simulink subsystem "ElectricalThermalSystem"  (R2024b)
settings: Solver=VariableStepAuto  StartTime=0.0  StopTime=10.0  RelTol=1e-3
undefined symbols (not defined in the file): EnvAirTemp, PlantThrEstCmpPwr, PlntThrAirBpt, PlntThrAirCond, PlntThrAirCp, PlntThrAirCpBpt, PlntThrAirPrand, PlntThrAirRho, PlntThrAirVisc, PlntThrBattDCFlwRatio, PlntThrBattJacLen, PlntThrChArea, PlntThrChDia, PlntThrCoolCond, PlntThrCoolCp, PlntThrCoolCpBpt, PlntThrCoolPrand, PlntThrCoolRho, PlntThrCoolVisc, PlntThrDCJacLen, PlntThrEMJacLen, PlntThrEstCOPLut, PlntThrEstDTLut, PlntThrHeaterMaxPwr, PlntThrPmpDisp, PlntThrPmpHeadP, PlntThrPmpMaxSpd, PlntThrPmpMechEff, PlntThrPmpVolEff, PlntThrRadAirArea, PlntThrRadAirDh, PlntThrRadFanAreaFlw, PlntThrRadFlwCoef, PlntThrRadGapHeight, PlntThrRadLength, PlntThrRadNTubes, PlntThrRadTubeDh, PlntThrRadTubeHeight, PlntThrRadWidth
libraries: autolibutils x45
(part 1 of 4)
settings Model: ModifiedByFormat=The MathWorks, Inc.  Creator=The MathWorks, Inc.  LastModifiedBy=The MathWorks, Inc.
settings RTWCC: GPUComputeCapability=3.5  LargeConstantGeneration=WriteOnlyDNNConstantsToDataFiles

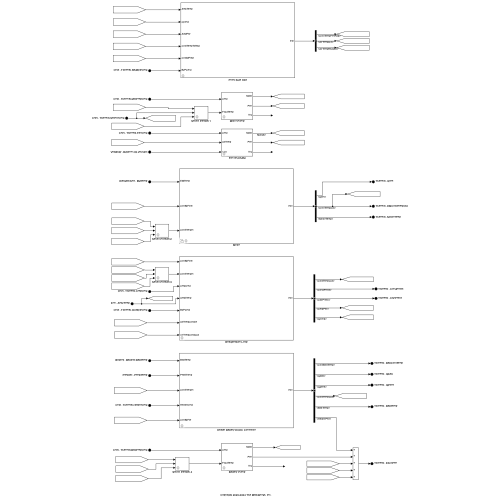
[thumbnail: Simulink's stored preview of the top-level diagram]
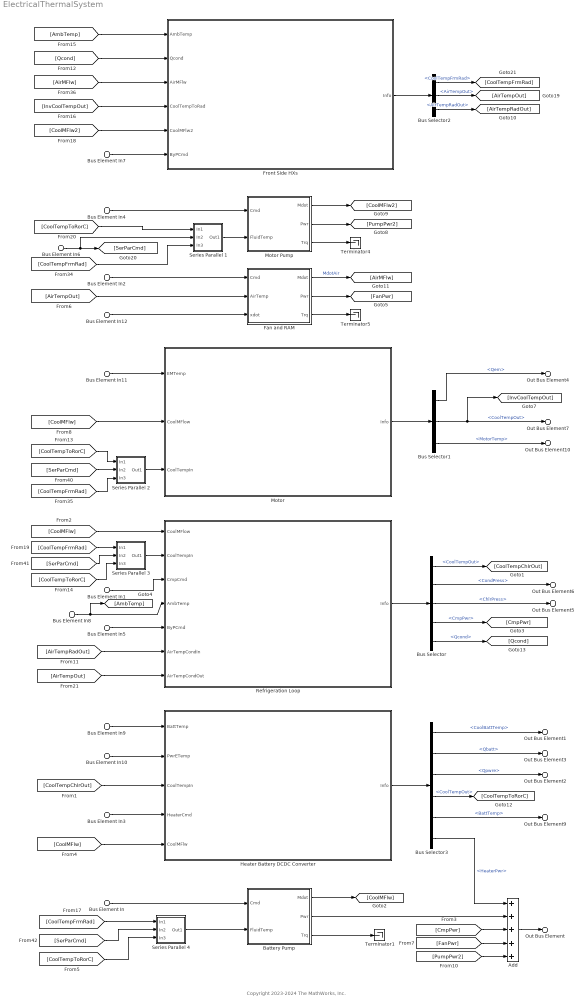
== system ElectricalThermalSystem ==
  note: Copyright 2023-2024 The MathWorks, Inc.
  Bus Element In : Inport  PortName=Cntrl  Element=Thermal.BattPmpCmd
  Bus Element In1 : Inport  PortName=Cntrl  Element=Thermal.CmpCmd
  Bus Element In2 : Inport  PortName=Cntrl  Element=Thermal.FanCmd
  Bus Element In3 : Inport  PortName=Cntrl  Element=Thermal.HeaterCmd
  Bus Element In4 : Inport  PortName=Cntrl  Element=Thermal.MotPmpCmd
  Bus Element In5 : Inport  PortName=Cntrl  Element=Thermal.ChlrByPCmd
  Bus Element In6 : Inport  PortName=Cntrl  Element=Thermal.SerParCmd
  Bus Element In7 : Inport  PortName=Cntrl  Element=Thermal.RadByPCmd
  Bus Element In8 : Inport  Port=2  PortName=Env  Element=AmbTemp
  Bus Element In9 : Inport  Port=3  PortName=Battery  Element=BattInfo.BattTemp
  Bus Element In10 : Inport  Port=4  PortName=PwrElec  Element=PwrETemp
  Bus Element In11 : Inport  Port=5  PortName=ElecMachine  Element=EMTemp
  Bus Element In12 : Inport  Port=6  PortName=VehBody  Element=BdyFrm.Cg.Vel.xdot
  Add : Sum  Inputs=+++++
  Battery Pump : Subsystem  mask{DispAng=PlntThrPmpDisp, MaxSpd=PlntThrPmpMaxSpd, VolEff=PlntThrPmpVolEff, MechEff=PlntThrPmpMechEff, HeadP=PlntThrPmpHeadP}
      mask prompts: DispAng "Displacement per revolution, DispAng [L/rev]"; MaxSpd "Max angular speed, MaxSpd [rpm]"; VolEff "Volumetric efficiency, VolEff [-]"; MechEff "Mechanical efficiency, MechEff [-]"; HeadP "Pressure gain, HeadP [Pa]"
      mask TypeOptions DispAng: Displ_LperRev/Value
      mask TypeOptions MaxSpd: MaxSpd_rpm/Value
      mask TypeOptions VolEff: VolumetricEfficiency/Value
      mask TypeOptions MechEff: MechanicalEfficiency/Value
      mask TypeOptions HeadP: PressGain_Pa/Value
      mask DialogControl DescTextVar Prompt: Battery Pump
      mask DialogControl ParameterGroupVar Prompt: Description
      mask DialogControl Control2 Prompt: Calculates the coolant mass flow through the loop that includes the battery and estimates the power and torque required by the pump.
      mask DialogControl Control3 Prompt: The mass flow calculation is an approximation for a positive displacement device.
      mask DialogControl Control4 Prompt: Mflw = Density*DispAng*Omega*VolEff
      mask DialogControl Control5 Prompt: Where:
      mask DialogControl Control6 Prompt: Mflw: mass flow
      mask DialogControl Control7 Prompt: DispAng: displacement/rotation angle
      mask DialogControl Control8 Prompt: Omega: angular speed
      mask DialogControl Control9 Prompt: VolEff: volumetric efficiency
      mask DialogControl Control10 Prompt: Torque = DispAng*MechEff*HeadP
      mask DialogControl Control11 Prompt: Where:
      mask DialogControl Control12 Prompt: MechEng: mechanical efficiency
      mask DialogControl Control13 Prompt: HeadP: pressure gain, pressure out - pressure in
      mask DialogControl Control14 Prompt: Power = Torque*Omega
      mask DialogControl Container3 Prompt: Parameters
  Bus Selector : BusSelector  OutputSignals=CoolTempOut,CondPress,ChlrPress,CmpPwr,Qcond
  Bus Selector1 : BusSelector  OutputSignals=Qem,CoolTempOut,MotorTemp
  Bus Selector2 : BusSelector  OutputSignals=CoolTempFrmRad,AirTempOut,AirTempRadOut
  Bus Selector3 : BusSelector  OutputSignals=CoolBattTemp,Qbatt,Qpwre,CoolTempOut,BattTemp,HeaterPwr
  Fan and RAM : Subsystem  mask{DispAng=PlntThrPmpDisp, MaxSpd=PlntThrPmpMaxSpd, VolEff=PlntThrPmpVolEff, MechEff=PlntThrPmpMechEff, HeadP=PlntThrPmpHeadP}
      mask prompts: DispAng "Displacement per revolution, DispAng [L/rev]"; MaxSpd "Max angular speed, MaxSpd [rpm]"; VolEff "Volumetric efficiency, VolEff [-]"; MechEff "Mechanical efficiency, MechEff [-]"; HeadP "Pressure gain, HeadP [Pa]"
      mask TypeOptions DispAng: Displ_LperRev/Value
      mask TypeOptions MaxSpd: MaxSpd_rpm/Value
      mask TypeOptions VolEff: VolumetricEfficiency/Value
      mask TypeOptions MechEff: MechanicalEfficiency/Value
      mask TypeOptions HeadP: PressGain_Pa/Value
      mask DialogControl DescTextVar Prompt: Fan and Ram
      mask DialogControl ParameterGroupVar Prompt: Description
      mask DialogControl Control2 Prompt: Calculates the air mass flow through the radiator and the condenser (Front Side HXs).
      mask DialogControl Control3 Prompt: The mass flow calculation is the sum of: (1) an approximation for a positive displacement device and (2) the ram effect. Estimates the power and torque required by the fan.
      mask DialogControl Control4 Prompt: Mflw = Density*DispAng*Omega*VolEff + Density*xdot*Ar*Crf
      mask DialogControl Control5 Prompt: Where:
      mask DialogControl Control6 Prompt: Mflw: mass flow
      mask DialogControl Control7 Prompt: DispAng: displacement/rotation angle
      mask DialogControl Control8 Prompt: Omega: angular speed
      mask DialogControl Control9 Prompt: VolEff: volumetric efficiency
      mask DialogControl Control15 Prompt: xdot: vehicle speed
      mask DialogControl Control16 Prompt: Ar: radiator fan area
      mask DialogControl Control17 Prompt: Crf: radiator flow coefficient
      mask DialogControl Control10 Prompt: Torque = DispAng*MechEff*HeadP
      mask DialogControl Control11 Prompt: Where:
      mask DialogControl Control12 Prompt: MechEng: mechanical efficiency
      mask DialogControl Control13 Prompt: HeadP: pressure gain, pressure out - pressure in
      mask DialogControl Control14 Prompt: Power = Torque*Omega
      mask DialogControl Container3 Prompt: Parameters
  Front Side HXs : Subsystem
      mask DialogControl Control1 Prompt: Front Side Heat Exchangers
      mask DialogControl Container2 Prompt: Description
      mask DialogControl Control16 Prompt: Contains the radiator (upstream) and the condenser.
      mask DialogControl Control2 Prompt: Inputs
      mask DialogControl Control3 Prompt: Env: bus containing ambient temperature signal.
      mask DialogControl Control4 Prompt: Qcond: heat dissipated by the condenser, from Refrigeration Loop subsystem.
      mask DialogControl Control5 Prompt: AirMFlw: air mass flow through (both) condenser and radiator, from Fan and Ram subsystem.
      mask DialogControl Control6 Prompt: InvCoolTempOut: temperature of the coolant coming out from the hottest electrical component (EMs), from Motor subsystem.
      mask DialogControl Control7 Prompt: CoolMFlw2: coolant mass flow from the loop that includes the EMs, from Motor Pump subsystem.
      mask DialogControl Control9 Prompt: RadByPCmd: control signal (0 or 1) to open or close the radiator bypass, 1 == bypassed radiator.
      mask DialogControl Control11 Prompt: Outputs
      mask DialogControl Control12 Prompt: CoolTempFrmRad: coolant temperature leaving the radiator.
      mask DialogControl Control13 Prompt: AirTempOut: air temperature leaving the condenser.
      mask DialogControl Control15 Prompt: AirTempRadOut: air temperature leaving the radiator (entering the condenser).
  Heater Battery DCDC Converter : Subsystem
      mask DialogControl DescTextVar Prompt: Heater Battery DCDC Converter
      mask DialogControl ParameterGroupVar Prompt: Description
      mask DialogControl Control2 Prompt: The DC-DC converter and the battery heat transfer is assumed to happen in cooling jackets. The two branches, (1) DC-DC Converter and (2) the battery heater (upstream) the battery itself are arranged in parallel.
  Motor : Subsystem  Variant=on
      mask DialogControl DescTextVar Prompt: Motor
      mask DialogControl ParameterGroupVar Prompt: Description
      mask DialogControl Control2 Prompt: The cooling of the electric machine(s) [EM(s)] is estimated with cooling jackets connected to each EM and arranged in series. The variant subsystem will choose the proper variant (1,2,3 or 4 EMs) according to the number of EMs (defined by the parameter PlntEMNum).
  Motor Pump : Subsystem  mask{DispAng=PlntThrPmpDisp, MaxSpd=PlntThrPmpMaxSpd, VolEff=PlntThrPmpVolEff, MechEff=PlntThrPmpMechEff, HeadP=PlntThrPmpHeadP}
      mask prompts: DispAng "Displacement per revolution, DispAng [L/rev]"; MaxSpd "Max angular speed, MaxSpd [rpm]"; VolEff "Volumetric efficiency, VolEff [-]"; MechEff "Mechanical efficiency, MechEff [-]"; HeadP "Pressure gain, HeadP [Pa]"
      mask TypeOptions DispAng: Displ_LperRev/Value
      mask TypeOptions MaxSpd: MaxSpd_rpm/Value
      mask TypeOptions VolEff: VolumetricEfficiency/Value
      mask TypeOptions MechEff: MechanicalEfficiency/Value
      mask TypeOptions HeadP: PressGain_Pa/Value
      mask DialogControl DescTextVar Prompt: Motor Pump
      mask DialogControl ParameterGroupVar Prompt: Description
      mask DialogControl Control2 Prompt: Calculates the coolant mass flow through the loop that includes the electric machines and estimates the power and torque required by the pump.
      mask DialogControl Control3 Prompt: The mass flow calculation is an approximation for a positive displacement device.
      mask DialogControl Control4 Prompt: Mflw = Density*DispAng*Omega*VolEff
      mask DialogControl Control5 Prompt: Where:
      mask DialogControl Control6 Prompt: Mflw: mass flow
      mask DialogControl Control7 Prompt: DispAng: displacement/rotation angle
      mask DialogControl Control8 Prompt: Omega: angular speed
      mask DialogControl Control9 Prompt: VolEff: volumetric efficiency
      mask DialogControl Control10 Prompt: Torque = DispAng*MechEff*HeadP
      mask DialogControl Control11 Prompt: Where:
      mask DialogControl Control12 Prompt: MechEng: mechanical efficiency
      mask DialogControl Control13 Prompt: HeadP: pressure gain, pressure out - pressure in
      mask DialogControl Control14 Prompt: Power = Torque*Omega
      mask DialogControl Container3 Prompt: Parameters
  Refrigeration Loop : Subsystem
      mask DialogControl DescTextVar Prompt: Refrigeration Loop
      mask DialogControl ParameterGroupVar Prompt: Description
      mask DialogControl Control2 Prompt: A simple reduced order model is implemented inside this subsystem, in place of a two-phase physics-based model of the refrigeration cycle. Specific outcomes are the chiller and condenser heat-flow rates and the compressor power.
      mask DialogControl Control3 Prompt: The outlet (refrigerant) pressure of the condenser and the chiller are also estimated and will be used as inputs by the controller.
  Series Parallel 1 : Subsystem
      mask DialogControl DescTextVar Prompt: Series Parallel
      mask DialogControl ParameterGroupVar Prompt: Description
      mask DialogControl Control2 Prompt: The Series Parallel switch re-routes signals configuring the system to operate in series or in parallel.
      mask DialogControl Control3 Prompt: Command == 1: Series configuration.
      mask DialogControl Control4 Prompt: Command == 0: Parallel configuration.
      mask DialogControl Control5 Prompt: Series configuration connection sequence: Radiator -> Battery Pump -> Refrigeration Loop (usually bypassed) -> [Battery Heater -> Battery and DC-DC converter in parallel] -> Motor Pump -> Motor(s) -> Radiator. The Radiator can be bypassed.
      mask DialogControl Control6 Prompt: Parallel configuration connection sequence: two circuits.
      mask DialogControl Control7 Prompt: Circuit 1: Radiator -> Motor Pump -> Motor(s) -> Radiator. The Radiator can be bypassed.
      mask DialogControl Control8 Prompt: Circuit 2: Battery Pump -> Refrigeration Loop -> [Battery Heater (off) -> Battery and DC-DC converter in parallel] -> Battery Pump.
  Series Parallel 2 : Subsystem
      mask DialogControl DescTextVar Prompt: Series Parallel
      mask DialogControl ParameterGroupVar Prompt: Description
      mask DialogControl Control2 Prompt: The Series Parallel switch re-routes signals configuring the system to operate in series or in parallel.
      mask DialogControl Control3 Prompt: Command == 1: Series configuration.
      mask DialogControl Control4 Prompt: Command == 0: Parallel configuration.
      mask DialogControl Control5 Prompt: Series configuration connection sequence: Radiator -> Battery Pump -> Refrigeration Loop (usually bypassed) -> [Battery Heater -> Battery and DC-DC converter in parallel] -> Motor Pump -> Motor(s) -> Radiator. The Radiator can be bypassed.
      mask DialogControl Control6 Prompt: Parallel configuration connection sequence: two circuits.
      mask DialogControl Control7 Prompt: Circuit 1: Radiator -> Motor Pump -> Motor(s) -> Radiator. The Radiator can be bypassed.
      mask DialogControl Control8 Prompt: Circuit 2: Battery Pump -> Refrigeration Loop -> [Battery Heater (off) -> Battery and DC-DC converter in parallel] -> Battery Pump.
  Series Parallel 3 : Subsystem
      mask DialogControl DescTextVar Prompt: Series Parallel
      mask DialogControl ParameterGroupVar Prompt: Description
      mask DialogControl Control2 Prompt: The Series Parallel switch re-routes signals configuring the system to operate in series or in parallel.
      mask DialogControl Control3 Prompt: Command == 1: Series configuration.
      mask DialogControl Control4 Prompt: Command == 0: Parallel configuration.
      mask DialogControl Control5 Prompt: Series configuration connection sequence: Radiator -> Battery Pump -> Refrigeration Loop (usually bypassed) -> [Battery Heater -> Battery and DC-DC converter in parallel] -> Motor Pump -> Motor(s) -> Radiator. The Radiator can be bypassed.
      mask DialogControl Control6 Prompt: Parallel configuration connection sequence: two circuits.
      mask DialogControl Control7 Prompt: Circuit 1: Radiator -> Motor Pump -> Motor(s) -> Radiator. The Radiator can be bypassed.
      mask DialogControl Control8 Prompt: Circuit 2: Battery Pump -> Refrigeration Loop -> [Battery Heater (off) -> Battery and DC-DC converter in parallel] -> Battery Pump.
  Series Parallel 4 : Subsystem
      mask DialogControl DescTextVar Prompt: Series Parallel
      mask DialogControl ParameterGroupVar Prompt: Description
      mask DialogControl Control2 Prompt: The Series Parallel switch re-routes signals configuring the system to operate in series or in parallel.
      mask DialogControl Control3 Prompt: Command == 1: Series configuration.
      mask DialogControl Control4 Prompt: Command == 0: Parallel configuration.
      mask DialogControl Control5 Prompt: Series configuration connection sequence: Radiator -> Battery Pump -> Refrigeration Loop (usually bypassed) -> [Battery Heater -> Battery and DC-DC converter in parallel] -> Motor Pump -> Motor(s) -> Radiator. The Radiator can be bypassed.
      mask DialogControl Control6 Prompt: Parallel configuration connection sequence: two circuits.
      mask DialogControl Control7 Prompt: Circuit 1: Radiator -> Motor Pump -> Motor(s) -> Radiator. The Radiator can be bypassed.
      mask DialogControl Control8 Prompt: Circuit 2: Battery Pump -> Refrigeration Loop -> [Battery Heater (off) -> Battery and DC-DC converter in parallel] -> Battery Pump.
  Terminator1 : Terminator
  Terminator4 : Terminator
  Terminator5 : Terminator
  Out Bus Element7 : Outport  PortName=Thermal  Element=EMCoolTempOut
  Out Bus Element9 : Outport  PortName=Thermal  Element=BattTemp
  Out Bus Element10 : Outport  PortName=Thermal  Element=MotorTemp
  Out Bus Element6 : Outport  PortName=Thermal  Element=CondPress
  Out Bus Element : Outport  PortName=Thermal  Element=EAccPwr
  Out Bus Element1 : Outport  PortName=Thermal  Element=BattCoolTemp
  Out Bus Element3 : Outport  PortName=Thermal  Element=Qbatt
  Out Bus Element2 : Outport  PortName=Thermal  Element=Qpwre
  Out Bus Element4 : Outport  PortName=Thermal  Element=Qem
  Out Bus Element5 : Outport  PortName=Thermal  Element=ChlrPress
  wires:
  [CoolTempFrmRad] -> Series Parallel 1/3(In3)
  [CoolTempToRorC] -> Series Parallel 1/1(In1)
  [CoolTempToRorC] -> Series Parallel 4/3(In3)
  [CoolTempFrmRad] -> Series Parallel 4/1(In1)
  [CoolTempFrmRad] -> Series Parallel 2/3(In3)
  [CoolTempToRorC] -> Series Parallel 2/1(In1)
  [CoolTempToRorC] -> Series Parallel 3/3(In3)
  [CoolTempFrmRad] -> Series Parallel 3/1(In1)
  Bus Selector3/6 -> Add/1  "<HeaterPwr>"
  Battery Pump/2(Pwr) -> Add/2
  [CmpPwr] -> Add/3
  [FanPwr] -> Add/4
  [PumpPwr2] -> Add/5
  Bus Selector3/5 -> Out Bus Element9/1  "<BattTemp>"
  Bus Selector1/3 -> Out Bus Element10/1  "<MotorTemp>"
  Bus Selector/1 -> [CoolTempChlrOut]  "<CoolTempOut>"
  Bus Selector2/1 -> [CoolTempFrmRad]  "<CoolTempFrmRad>"
  [CoolMFlw2] -> Front Side HXs/5(CoolMFlw2)
  Bus Element In6/1 -> Series Parallel 1/2(In2), [SerParCmd]
  [SerParCmd] -> Series Parallel 3/2(In2)
  [SerParCmd] -> Series Parallel 4/2(In2)
  [SerParCmd] -> Series Parallel 2/2(In2)
  Bus Selector2/2 -> [AirTempOut]  "<AirTempOut>"
  Front Side HXs/1(Info) -> Bus Selector2/1
  [InvCoolTempOut] -> Front Side HXs/4(CoolTempToRad)
  [AirMFlw] -> Front Side HXs/3(AirMFlw)
  [Qcond] -> Front Side HXs/2(Qcond)
  [AmbTemp] -> Front Side HXs/1(AmbTemp)
  Refrigeration Loop/1(Info) -> Bus Selector/1
  Bus Selector/5 -> [Qcond]  "<Qcond>"
  Motor Pump/1(Mdot) -> [CoolMFlw2]
  Motor Pump/2(Pwr) -> [PumpPwr2]
  Motor Pump/3(Trq) -> Terminator4/1
  Bus Element In4/1 -> Motor Pump/1(Cmd)
  Bus Selector1/2 -> [InvCoolTempOut], Out Bus Element7/1  "<CoolTempOut>"
  Bus Selector1/1 -> Out Bus Element4/1  "<Qem>"
  Fan and RAM/3(Trq) -> Terminator5/1
  Fan and RAM/2(Pwr) -> [FanPwr]
  Fan and RAM/1(Mdot) -> [AirMFlw]  "MdotAir"
  Bus Element In2/1 -> Fan and RAM/1(Cmd)
  [AirTempOut] -> Fan and RAM/2(AirTemp)
  [CoolMFlw] -> Heater Battery DCDC Converter/5(CoolMFlw)
  Add/1 -> Out Bus Element/1
  Bus Selector/3 -> Out Bus Element5/1  "<ChlrPress>"
  Bus Selector/2 -> Out Bus Element6/1  "<CondPress>"
  Bus Selector/4 -> [CmpPwr]  "<CmpPwr>"
  [CoolTempChlrOut] -> Heater Battery DCDC Converter/3(CoolTempIn)
  Bus Element In1/1 -> Refrigeration Loop/3(CmpCmd)
  [CoolMFlw] -> Refrigeration Loop/1(CoolMFlow)
  Bus Selector3/4 -> [CoolTempToRorC]  "<CoolTempOut>"
  Bus Selector3/3 -> Out Bus Element2/1  "<Qpwre>"
  Bus Selector3/2 -> Out Bus Element3/1  "<Qbatt>"
  Bus Selector3/1 -> Out Bus Element1/1  "<CoolBattTemp>"
  Heater Battery DCDC Converter/1(Info) -> Bus Selector3/1
  Bus Element In3/1 -> Heater Battery DCDC Converter/4(HeaterCmd)
  Battery Pump/3(Trq) -> Terminator1/1
  Battery Pump/1(Mdot) -> [CoolMFlw]
  Bus Element In/1 -> Battery Pump/1(Cmd)
  Bus Element In7/1 -> Front Side HXs/6(ByPCmd)
  Bus Element In5/1 -> Refrigeration Loop/5(ByPCmd)
  Bus Selector2/3 -> [AirTempRadOut]  "<AirTempRadOut>"
  [AirTempRadOut] -> Refrigeration Loop/6(AirTempCondIn)
  [AirTempOut] -> Refrigeration Loop/7(AirTempCondOut)
  Bus Element In8/1 -> [AmbTemp], Refrigeration Loop/4(AmbTemp)
  Bus Element In12/1 -> Fan and RAM/3(xdot)
  Bus Element In11/1 -> Motor/1(EMTemp)
  [CoolMFlw] -> Motor/2(CoolMFlow)
  Series Parallel 2/1(Out1) -> Motor/3(CoolTempIn)
  Motor/1(Info) -> Bus Selector1/1
  Series Parallel 1/1(Out1) -> Motor Pump/2(FluidTemp)
  Series Parallel 3/1(Out1) -> Refrigeration Loop/2(CoolTempIn)
  Series Parallel 4/1(Out1) -> Battery Pump/2(FluidTemp)
  Bus Element In10/1 -> Heater Battery DCDC Converter/2(PwrETemp)
  Bus Element In9/1 -> Heater Battery DCDC Converter/1(BattTemp)

== system ElectricalThermalSystem/Battery Pump ==
  Cmd : Inport
  FluidTemp : Inport  Port=2
  Density : Lookup_n-D  NumberOfTableDimensions=1  BreakpointsForDimension1=PlntThrCoolCpBpt  Table=PlntThrCoolRho  ExtrapMethod=Clip  UseLastTableValue=on  InternalRulePriority=Speed  RndMeth=Simplest
  Displ_LperRev : Constant  Value=DispAng  SampleTime=-1
  Gain : Gain  Gain=2*pi/60
  Gain1 : Gain  Gain=1/(1000*2*pi)
  LPF with IC1 : Subsystem  mask{wc=100, InitCond=0, dataType=off}
      mask prompts: wc "Cutoff frequency, wc [rad/s]"; InitCond "Initial condition, InitCond [same as u]"; dataType "Enforce same input data type"
      mask TypeOptions wc: Cont LPF IC/wc
      mask TypeOptions InitCond: Initial Condition/Value
      mask TypeOptions dataType: Cont LPF IC/dataType
  MaxSpd_rpm : Constant  Value=MaxSpd  SampleTime=-1
  MechanicalEfficiency : Constant  Value=MechEff  SampleTime=-1
  PressGain_Pa : Constant  Value=HeadP  SampleTime=-1
  Product : Product  Inputs=4
  Product1 : Product  Inputs=3
  Product2 : Product
  Product7 : Product
  Saturation : Saturate  UpperLimit=inf  LowerLimit=0
  VolumetricEfficiency : Constant  Value=VolEff  SampleTime=-1
  Mdot : Outport
  Pwr : Outport  Port=2
  Trq : Outport  Port=3
  wires:
  Product2/1 -> Pwr/1
  Cmd/1 -> LPF with IC1/1(u)
  Product/1 -> Saturation/1
  Gain1/1 -> Product/2, Product1/1
  Product1/1 -> Product2/2, Trq/1
  PressGain_Pa/1 -> Product1/3
  [Spd] -> Product2/1
  MechanicalEfficiency/1 -> Product1/2
  [VolEff] -> Product/4
  [Spd] -> Product/3
  Product7/1 -> [Spd]
  Displ_LperRev/1 -> Gain1/1
  Gain/1 -> Product7/1
  MaxSpd_rpm/1 -> Gain/1
  Density/1 -> Product/1
  VolumetricEfficiency/1 -> [VolEff]
  FluidTemp/1 -> Density/1
  LPF with IC1/1(y) -> Product7/2
  Saturation/1 -> Mdot/1

== system ElectricalThermalSystem/Fan and RAM ==
  Cmd : Inport
  AirTemp : Inport  Port=2
  xdot : Inport  Port=3
  Add : Sum
  Density : Lookup_n-D  NumberOfTableDimensions=1  BreakpointsForDimension1=PlntThrAirBpt  Table=PlntThrAirRho  ExtrapMethod=Clip  UseLastTableValue=on  InternalRulePriority=Speed  RndMeth=Simplest
  Displ_LperRev : Constant  Value=DispAng  SampleTime=-1
  Gain : Gain  Gain=PlntThrRadFanAreaFlw*PlntThrRadFlwCoef
  Gain1 : Gain  Gain=2*pi/60
  Gain2 : Gain  Gain=1/(1000*2*pi)
  LPF with IC1 : Subsystem  mask{wc=100, InitCond=0, dataType=off}
      mask prompts: wc "Cutoff frequency, wc [rad/s]"; InitCond "Initial condition, InitCond [same as u]"; dataType "Enforce same input data type"
      mask TypeOptions wc: Cont LPF IC/wc
      mask TypeOptions InitCond: Initial Condition/Value
      mask TypeOptions dataType: Cont LPF IC/dataType
  MaxSpd_rpm : Constant  Value=MaxSpd  SampleTime=-1
  MechanicalEfficiency : Constant  Value=MechEff  SampleTime=-1
  PressGain_Pa : Constant  Value=HeadP  SampleTime=-1
  Product : Product  Inputs=3
  Product1 : Product  Inputs=3
  Product2 : Product
  Product4 : Product
  Product7 : Product
  Saturation : Saturate  UpperLimit=inf  LowerLimit=0
  VolumetricEfficiency : Constant  Value=VolEff  SampleTime=-1
  Mdot : Outport
  Pwr : Outport  Port=2
  Trq : Outport  Port=3
  wires:
  Gain/1 -> Add/1
  Add/1 -> Product4/2
  [Spd] -> Product/2
  [VolEff] -> Product/3
  Product2/1 -> Pwr/1
  Cmd/1 -> LPF with IC1/1(u)
  Gain2/1 -> Product/1, Product1/1
  Product1/1 -> Product2/2, Trq/1
  PressGain_Pa/1 -> Product1/3
  [Spd] -> Product2/1
  MechanicalEfficiency/1 -> Product1/2
  Product7/1 -> [Spd]
  Displ_LperRev/1 -> Gain2/1
  Gain1/1 -> Product7/1
  MaxSpd_rpm/1 -> Gain1/1
  Density/1 -> Product4/1
  VolumetricEfficiency/1 -> [VolEff]
  xdot/1 -> Gain/1
  Product/1 -> Add/2  "FanAir"
  AirTemp/1 -> Density/1
  LPF with IC1/1(y) -> Product7/2
  Saturation/1 -> Mdot/1
  Product4/1 -> Saturation/1

== system ElectricalThermalSystem/Front Side HXs ==
  AmbTemp : Inport
  Qcond : Inport  Port=2
  AirMFlw : Inport  Port=3
  CoolTempToRad : Inport  Port=4
  CoolMFlw2 : Inport  Port=5
  ByPCmd : Inport  Port=6
  Condenser : Subsystem
      mask DialogControl Control1 Prompt: Condenser
      mask DialogControl Container2 Prompt: Description
      mask DialogControl Control2 Prompt: Calculates the increase in air temperature through the condenser due to the refrigerant heat dissipation.
      mask DialogControl Control3 Prompt: Q = mdot*Cp*(Tout-Tin)
      mask DialogControl Control4 Prompt: Where:
      mask DialogControl Control5 Prompt: Q: heat flow
      mask DialogControl Control6 Prompt: mdot: mass flow
      mask DialogControl Control7 Prompt: Cp: heat capacity
      mask DialogControl Control8 Prompt: Tout: temperature out
      mask DialogControl Control9 Prompt: Tin: temperature in
  Radiator : Subsystem
      mask DialogControl Control1 Prompt: Radiator
      mask DialogControl Container2 Prompt: Description
      mask DialogControl Control2 Prompt: The outlet temperatures for air and coolant are not known, therefore, the heat exchanger effectiveness is utilized as an estimation method.
      mask DialogControl Control3 Prompt: The heat exchanger effectiveness is defined as the ratio of the actual rate of heat to the maximum possible.
      mask DialogControl Control4 Prompt: Effectiveness can be expressed in terms of dimensionless parameters, the heat capacity rate ratio (Cmin/Cmax) and the ratio of the overall conductance to the smaller heat capacity rate (UA/Cmin), also called Number of Heat-transfer Units (NTU).
      mask DialogControl Control5 Prompt: Inside subsystem masks describe the method derivation:
      mask DialogControl Control6 Prompt: Subsystem NTU and Dimensions: UA and NTU
      mask DialogControl Control7 Prompt: Subsystem Effectiveness: Effectiveness
      mask DialogControl Control8 Prompt: Subsystem Heat Capacity Rate: Cmin, Cmax, Cmin/Cmax
      mask DialogControl Control9 Prompt: Subsystems Air Temperature and Coolant Temperature estimate the temperatures for air and coolant leaving the radiator, respectively, as well as the heat rate.
  Out Bus Element : Outport  PortName=Info  Element=CoolTempFrmRad
  Out Bus Element1 : Outport  PortName=Info  Element=AirTempOut
  Out Bus Element2 : Outport  PortName=Info  Element=Qrad
  Out Bus Element3 : Outport  PortName=Info  Element=AirTempRadOut
  wires:
  AirMFlw/1 -> Radiator/4(MassFlow2), [AirMassFlw]  "AirMassFlow"
  Qcond/1 -> Condenser/1(Qcond)
  Condenser/1(AirTempOut) -> Out Bus Element1/1
  Radiator/3(AirTempOut) -> Condenser/3(AirTempRadOut), Out Bus Element3/1
  CoolTempToRad/1 -> Radiator/1(CoolTempToRad)
  AmbTemp/1 -> Radiator/2(AmbTemp)
  CoolMFlw2/1 -> Radiator/3(CoolMFlw)
  ByPCmd/1 -> Radiator/5(ByPCmd)
  Radiator/1(CoolTempFrmRad) -> Out Bus Element/1
  Radiator/2(Qrad) -> Out Bus Element2/1
  [AirMassFlw] -> Condenser/2(AirMassFlow)

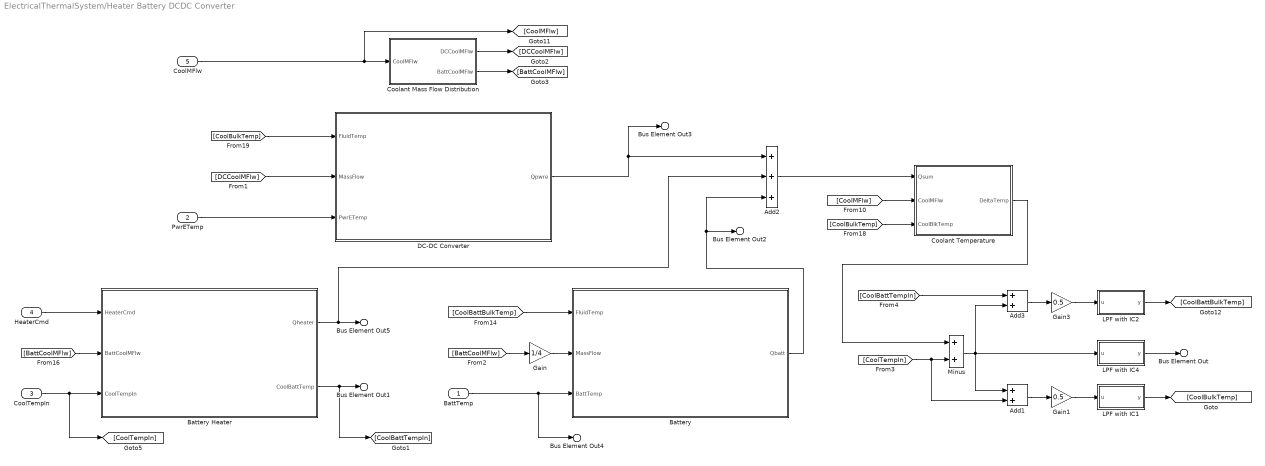
== system ElectricalThermalSystem/Heater Battery DCDC Converter ==
  BattTemp : Inport
  PwrETemp : Inport  Port=2
  CoolTempIn : Inport  Port=3
  HeaterCmd : Inport  Port=4
  CoolMFlw : Inport  Port=5
  Add1 : Sum
  Add2 : Sum  Inputs=+++
  Add3 : Sum
  Battery : Subsystem  mask{JacArea=PlntThrChArea, JacDia=PlntThrChDia, JacLen=PlntThrBattJacLen, JacHtArea=PlntThrBattJacLen*pi*PlntThrChDia}
      mask prompts: JacArea "Jacket cross section area, JacArea [m^2]"; JacDia "Jacket hydraulic diameter, JacDia [m]"; JacLen "Jacket length, JacLen [m]"; JacHtArea "Jacket heat transfer area, JacHtArea [m^2]"
      mask TypeOptions JacArea: Constant7/Value
      mask TypeOptions JacDia: Constant6/Value
      mask TypeOptions JacLen: Constant8/Value
      mask TypeOptions JacHtArea: Constant3/Value
      mask DialogControl DescTextVar Prompt: Battery
      mask DialogControl ParameterGroupVar Prompt: Description
      mask DialogControl Control2 Prompt: The cooling of the battery is estimated with a cooling jacket. Dimensions must be set in order to estimate its convective heat transfer coefficient (HTC) and heat-flow rate.
      mask DialogControl Container3 Prompt: Parameters
  Battery Heater : Subsystem  mask{HtPwr=PlntThrHeaterMaxPwr}
      mask prompts: HtPwr "Maximum battery heater power, Gain [W]"
      mask TypeOptions HtPwr: Max Heat/Gain
      mask DialogControl DescTextVar Prompt: Battery Heater
      mask DialogControl ParameterGroupVar Prompt: Description
      mask DialogControl Control2 Prompt: Maximum battery heater power times heater control signal (0 to 1) equals heat-flow rate.
      mask DialogControl Container3 Prompt: Parameters
  Coolant Mass Flow Distribution : Subsystem  mask{MFlwRt=PlntThrBattDCFlwRatio}
      mask prompts: MFlwRt "Battery / DC-DC converter flow ratio, MFlwRt [-]"
      mask TypeOptions MFlwRt: Gain2/Gain
      mask DialogControl DescTextVar Prompt: Coolant Mass Flow Distribution
      mask DialogControl ParameterGroupVar Prompt: Description
      mask DialogControl Control2 Prompt: The battery and the DC-DC converter cooling is in parallel, therefore an estimate of the ratio of mass flow to the battery over the flow through the DC-DC converter must be entered.
      mask DialogControl Container3 Prompt: Parameters
  Coolant Temperature : Subsystem
      mask DialogControl DescTextVar Prompt: Coolant Temperature
      mask DialogControl ParameterGroupVar Prompt: Description
      mask DialogControl Control2 Prompt: Calculates the change in coolant temperature.
      mask DialogControl Control3 Prompt: Q = mdot*Cp*DeltaTemp
      mask DialogControl Control4 Prompt: Where:
      mask DialogControl Control5 Prompt: Q: heat-flow rate
      mask DialogControl Control6 Prompt: mdot: mass flow
      mask DialogControl Control7 Prompt: Cp: heat capacity
      mask DialogControl Control10 Prompt: DeltaTemp = Tout - Tin
      mask DialogControl Control8 Prompt: Tout: coolant temperature (outlet)
      mask DialogControl Control9 Prompt: Tin: coolant temperature (inlet)
  DC-DC Converter : Subsystem  mask{JacArea=PlntThrChArea, JacDia=PlntThrChDia, JacLen=PlntThrDCJacLen, JacHtArea=PlntThrDCJacLen*pi*PlntThrChDia}
      mask prompts: JacArea "Jacket cross section area, JacArea [m^2]"; JacDia "Jacket hydraulic diameter, JacDia [m]"; JacLen "Jacket length, JacLen [m]"; JacHtArea "Jacket heat transfer area, JacHtArea [m^2]"
      mask TypeOptions JacArea: Constant4/Value
      mask TypeOptions JacDia: Constant/Value
      mask TypeOptions JacLen: Constant5/Value
      mask TypeOptions JacHtArea: Constant2/Value
      mask DialogControl DescTextVar Prompt: DC-DC Converter
      mask DialogControl ParameterGroupVar Prompt: Description
      mask DialogControl Control2 Prompt: The cooling of the DC-DC converter is estimated with a cooling jacket. Dimensions must be set in order to estimate its convective heat transfer coefficient (HTC) and heat-flow rate.
      mask DialogControl Container3 Prompt: Parameters
  Gain : Gain  Gain=1/4
  Gain1 : Gain  Gain=0.5
  Gain3 : Gain  Gain=0.5
  LPF with IC1 : Subsystem  mask{wc=10, InitCond=EnvAirTemp, dataType=off}
      mask prompts: wc "Cutoff frequency, wc [rad/s]"; InitCond "Initial condition, InitCond [same as u]"; dataType "Enforce same input data type"
      mask TypeOptions wc: Cont LPF IC/wc
      mask TypeOptions InitCond: Initial Condition/Value
      mask TypeOptions dataType: Cont LPF IC/dataType
  LPF with IC2 : Subsystem  mask{wc=10, InitCond=EnvAirTemp, dataType=off}
      mask prompts: wc "Cutoff frequency, wc [rad/s]"; InitCond "Initial condition, InitCond [same as u]"; dataType "Enforce same input data type"
      mask TypeOptions wc: Cont LPF IC/wc
      mask TypeOptions InitCond: Initial Condition/Value
      mask TypeOptions dataType: Cont LPF IC/dataType
  LPF with IC4 : Subsystem  mask{wc=10, InitCond=EnvAirTemp, dataType=off}
      mask prompts: wc "Cutoff frequency, wc [rad/s]"; InitCond "Initial condition, InitCond [same as u]"; dataType "Enforce same input data type"
      mask TypeOptions wc: Cont LPF IC/wc
      mask TypeOptions InitCond: Initial Condition/Value
      mask TypeOptions dataType: Cont LPF IC/dataType
  Minus : Sum
  Bus Element Out : Outport  PortName=Info  Element=CoolTempOut
  Bus Element Out1 : Outport  PortName=Info  Element=CoolBattTemp
  Bus Element Out2 : Outport  PortName=Info  Element=Qbatt
  Bus Element Out3 : Outport  PortName=Info  Element=Qpwre
  Bus Element Out4 : Outport  PortName=Info  Element=BattTemp
  Bus Element Out5 : Outport  PortName=Info  Element=HeaterPwr
  wires:
  [CoolTempIn] -> Add1/2, Minus/2
  Minus/1 -> LPF with IC4/1(u), Add1/1, Add3/2
  Add3/1 -> Gain3/1
  CoolMFlw/1 -> [CoolMFlw], Coolant Mass Flow Distribution/1(CoolMFlw)
  CoolTempIn/1 -> [CoolTempIn], Battery Heater/3(CoolTempIn)
  Add1/1 -> Gain1/1
  Gain3/1 -> LPF with IC2/1(u)
  LPF with IC2/1(y) -> [CoolBattBulkTemp]
  Gain1/1 -> LPF with IC1/1(u)
  LPF with IC1/1(y) -> [CoolBulkTemp]
  LPF with IC4/1(y) -> Bus Element Out/1
  [BattCoolMFlw] -> Gain/1
  Coolant Mass Flow Distribution/1(DCCoolMFlw) -> [DCCoolMFlw]
  Coolant Mass Flow Distribution/2(BattCoolMFlw) -> [BattCoolMFlw]
  BattTemp/1 -> Battery/3(BattTemp), Bus Element Out4/1
  Battery/1(Qbatt) -> Add2/3, Bus Element Out2/1
  [CoolBattBulkTemp] -> Battery/1(FluidTemp)
  Gain/1 -> Battery/2(MassFlow)
  DC-DC Converter/1(Qpwre) -> Bus Element Out3/1, Add2/1
  [CoolBulkTemp] -> DC-DC Converter/1(FluidTemp)
  [DCCoolMFlw] -> DC-DC Converter/2(MassFlow)
  PwrETemp/1 -> DC-DC Converter/3(PwrETemp)
  HeaterCmd/1 -> Battery Heater/1(HeaterCmd)
  [BattCoolMFlw] -> Battery Heater/2(BattCoolMFlw)
  Add2/1 -> Coolant Temperature/1(Qsum)
  [CoolMFlw] -> Coolant Temperature/2(CoolMFlw)
  [CoolBulkTemp] -> Coolant Temperature/3(CoolBlkTemp)
  Coolant Temperature/1(DeltaTemp) -> Minus/1
  Battery Heater/2(CoolBattTemp) -> [CoolBattTempIn], Bus Element Out1/1
  [CoolBattTempIn] -> Add3/1
  Battery Heater/1(Qheater) -> Bus Element Out5/1, Add2/2

== system ElectricalThermalSystem/Motor ==
  EMTemp : Inport
  CoolMFlow : Inport  Port=2
  CoolTempIn : Inport  Port=3
  FourEMs : Subsystem  VariantControl=PlntEMNum == 4
  OneEM : Subsystem  VariantControl=PlntEMNum == 1
  ThreeEMs : Subsystem  VariantControl=PlntEMNum == 3
  TwoEMs : Subsystem  VariantControl=PlntEMNum == 2
  Info : Outport

== system ElectricalThermalSystem/Motor Pump ==
  Cmd : Inport
  FluidTemp : Inport  Port=2
  Density : Lookup_n-D  NumberOfTableDimensions=1  BreakpointsForDimension1=PlntThrCoolCpBpt  Table=PlntThrCoolRho  ExtrapMethod=Clip  UseLastTableValue=on  InternalRulePriority=Speed  RndMeth=Simplest
  Displ_LperRev : Constant  Value=DispAng  SampleTime=-1
  Gain : Gain  Gain=2*pi/60
  Gain1 : Gain  Gain=1/(1000*2*pi)
  LPF with IC1 : Subsystem  mask{wc=100, InitCond=0, dataType=off}
      mask prompts: wc "Cutoff frequency, wc [rad/s]"; InitCond "Initial condition, InitCond [same as u]"; dataType "Enforce same input data type"
      mask TypeOptions wc: Cont LPF IC/wc
      mask TypeOptions InitCond: Initial Condition/Value
      mask TypeOptions dataType: Cont LPF IC/dataType
  MaxSpd_rpm : Constant  Value=MaxSpd  SampleTime=-1
  MechanicalEfficiency : Constant  Value=MechEff  SampleTime=-1
  PressGain_Pa : Constant  Value=HeadP  SampleTime=-1
  Product : Product  Inputs=4
  Product1 : Product  Inputs=3
  Product2 : Product
  Product7 : Product
  Saturation : Saturate  UpperLimit=inf  LowerLimit=0
  VolumetricEfficiency : Constant  Value=VolEff  SampleTime=-1
  Mdot : Outport
  Pwr : Outport  Port=2
  Trq : Outport  Port=3
  wires:
  Product2/1 -> Pwr/1
  Cmd/1 -> LPF with IC1/1(u)
  Product/1 -> Saturation/1
  Gain1/1 -> Product/2, Product1/1
  Product1/1 -> Product2/2, Trq/1
  PressGain_Pa/1 -> Product1/3
  [Spd] -> Product2/1
  MechanicalEfficiency/1 -> Product1/2
  [VolEff] -> Product/4
  [Spd] -> Product/3
  Product7/1 -> [Spd]
  Displ_LperRev/1 -> Gain1/1
  Gain/1 -> Product7/1
  MaxSpd_rpm/1 -> Gain/1
  Density/1 -> Product/1
  VolumetricEfficiency/1 -> [VolEff]
  FluidTemp/1 -> Density/1
  LPF with IC1/1(y) -> Product7/2
  Saturation/1 -> Mdot/1

== system ElectricalThermalSystem/Refrigeration Loop ==
  CoolMFlow : Inport
  CoolTempIn : Inport  Port=2
  CmpCmd : Inport  Port=3
  AmbTemp : Inport  Port=4
  ByPCmd : Inport  Port=5
  AirTempCondIn : Inport  Port=6
  AirTempCondOut : Inport  Port=7
  Chiller Coolant Temperature : Subsystem
      mask DialogControl DescTextVar Prompt: Chiller Coolant Temperature
      mask DialogControl ParameterGroupVar Prompt: Description
      mask DialogControl Control2 Prompt: Calculates the change in coolant temperature through the chiller and adds it to the inlet temperature to calculate the outlet temperature.
      mask DialogControl Control3 Prompt: Q = mdot*Cp*(Tout-Tin)
      mask DialogControl Control4 Prompt: Where:
      mask DialogControl Control5 Prompt: Q: heat-flow rate
      mask DialogControl Control7 Prompt: mdot: mass flow
      mask DialogControl Control8 Prompt: Cp: heat capacity
      mask DialogControl Control10 Prompt: Tout: temperature (outlet)
      mask DialogControl Control9 Prompt: Tin: temperature (inlet)
  Chiller Pressure : Subsystem
      mask DialogControl DescTextVar Prompt: Chiller Pressure
      mask DialogControl ParameterGroupVar Prompt: Description
      mask DialogControl Control2 Prompt: The chiller refrigerant outlet pressure is estimated with tabulated empirical data.
      mask DialogControl Control3 Prompt: Pressure is assumed to depend (solely) on the difference in temperature of the coolant entering the chiller minus the temperature of the coolant leaving the chiller.
      mask DialogControl Control4 Prompt: The tabulated data resides in an LUT and must be calibrated to the specific refrigeration cycle.
      mask DialogControl Control5 Prompt: The pressure signal is used by the controller.
  Condenser Pressure : Subsystem
      mask DialogControl DescTextVar Prompt: Condenser Pressure
      mask DialogControl ParameterGroupVar Prompt: Description
      mask DialogControl Control5 Prompt: The condenser refrigerant outlet pressure is estimated with tabulated empirical data.
      mask DialogControl Control2 Prompt: Pressure is assumed to depend (solely) on the difference in temperature of the air leaving the condenser minus the temperature of the air entering the condenser.
      mask DialogControl Control3 Prompt: The tabulated data resides in an LUT and must be calibrated to the specific refrigeration cycle.
      mask DialogControl Control4 Prompt: The pressure signal is used by the controller.
  Heat-flow Rate and Power : Subsystem
      mask DialogControl DescTextVar Prompt: Heat-flow and Power
      mask DialogControl ParameterGroupVar Prompt: Description
      mask DialogControl Control2 Prompt: Heat-flow rates and power required by the refrigeration cycle are estimated by an empirical relation that resides in an LUT. It is based on the coefficient of performance (COP), which is defined as the ratio of the amount of heat-flow rate removed from the chiller to the amount of (compressor) power required to remove that heat.
      mask DialogControl Control3 Prompt: The COP is assumed to depend (solely) on the difference of the ambient temperature minus the coolant temperature entering the chiller. The COP tabulated data must be calibrated to the specific refrigeration cycle.
      mask DialogControl Control4 Prompt: COP times compressor power equals the heat-flow rate removed from the coolant in the chiller. This later, added to the compressor power, constitutes the heat-flow rate dissipated by the condenser.
  Out Bus Element : Outport  PortName=Info  Element=CoolTempOut
  Out Bus Element1 : Outport  PortName=Info  Element=CondPress
  Out Bus Element2 : Outport  PortName=Info  Element=ChlrPress
  Out Bus Element3 : Outport  PortName=Info  Element=CmpPwr
  Out Bus Element4 : Outport  PortName=Info  Element=Qcond
  wires:
  AirTempCondOut/1 -> Condenser Pressure/1(AirTempOut)
  AirTempCondIn/1 -> Condenser Pressure/2(AirTempIn)
  Condenser Pressure/1(CondPress) -> Out Bus Element1/1
  [CoolTempIn] -> Chiller Pressure/1(CoolTempIn)
  [CoolTempOut] -> Chiller Pressure/2(CoolTempOut)
  Chiller Pressure/1(ChlrPress) -> Out Bus Element2/1
  Chiller Coolant Temperature/1(CoolTOut) -> Out Bus Element/1, [CoolTempOut]
  [CoolTempOut] -> Chiller Coolant Temperature/2(CoolTempOut)
  CoolTempIn/1 -> [CoolTempIn], Chiller Coolant Temperature/3(CoolTempIn)
  CoolMFlow/1 -> Chiller Coolant Temperature/4(CoolMFlw)
  ByPCmd/1 -> Chiller Coolant Temperature/5(ByPCmd)
  AmbTemp/1 -> Heat-flow Rate and Power/1(AmbTemp)
  [CoolTempIn] -> Heat-flow Rate and Power/2(CoolTempIn)
  CmpCmd/1 -> Heat-flow Rate and Power/3(CmpCmd)
  Heat-flow Rate and Power/1(Qcond) -> Out Bus Element4/1
  Heat-flow Rate and Power/2(CmpPwr) -> Out Bus Element3/1
  Heat-flow Rate and Power/3(Qchiller) -> Chiller Coolant Temperature/1(Qchiller)

== system ElectricalThermalSystem/Series Parallel 1 ==
  In1 : Inport
  In2 : Inport  Port=2
  In3 : Inport  Port=3
  Series Parallel : Switch  Criteria=u2 > Threshold  Threshold=0.5  SaturateOnIntegerOverflow=off  InputSameDT=off
  Out1 : Outport
  wires:
  Series Parallel/1 -> Out1/1
  In1/1 -> Series Parallel/1
  In2/1 -> Series Parallel/2
  In3/1 -> Series Parallel/3

== system ElectricalThermalSystem/Series Parallel 2 ==
  In1 : Inport
  In2 : Inport  Port=2
  In3 : Inport  Port=3
  Series Parallel : Switch  Criteria=u2 > Threshold  Threshold=0.5  SaturateOnIntegerOverflow=off  InputSameDT=off
  Out1 : Outport
  wires:
  Series Parallel/1 -> Out1/1
  In1/1 -> Series Parallel/1
  In2/1 -> Series Parallel/2
  In3/1 -> Series Parallel/3

== system ElectricalThermalSystem/Series Parallel 3 ==
  In1 : Inport
  In2 : Inport  Port=2
  In3 : Inport  Port=3
  Series Parallel : Switch  Criteria=u2 > Threshold  Threshold=0.5  SaturateOnIntegerOverflow=off  InputSameDT=off
  Out1 : Outport
  wires:
  Series Parallel/1 -> Out1/1
  In1/1 -> Series Parallel/1
  In2/1 -> Series Parallel/2
  In3/1 -> Series Parallel/3

== system ElectricalThermalSystem/Series Parallel 4 ==
  In1 : Inport
  In2 : Inport  Port=2
  In3 : Inport  Port=3
  Series Parallel : Switch  Criteria=u2 > Threshold  Threshold=0.5  SaturateOnIntegerOverflow=off  InputSameDT=off
  Out1 : Outport
  wires:
  Series Parallel/1 -> Out1/1
  In1/1 -> Series Parallel/1
  In2/1 -> Series Parallel/2
  In3/1 -> Series Parallel/3

== system ElectricalThermalSystem/Battery Pump/LPF with IC1 ==
  u : Inport
  Cont LPF IC : autolibutils/Cont LPF IC  wc=wc  aMode=1  dataType=off
  Initial Condition : Constant  Value=InitCond  SampleTime=-1
  y : Outport
  wires:
  Initial Condition/1 -> Cont LPF IC/2
  u/1 -> Cont LPF IC/1
  Cont LPF IC/1 -> y/1

== system ElectricalThermalSystem/Fan and RAM/LPF with IC1 ==
  u : Inport
  Cont LPF IC : autolibutils/Cont LPF IC  wc=wc  aMode=1  dataType=off
  Initial Condition : Constant  Value=InitCond  SampleTime=-1
  y : Outport
  wires:
  Initial Condition/1 -> Cont LPF IC/2
  u/1 -> Cont LPF IC/1
  Cont LPF IC/1 -> y/1

== system ElectricalThermalSystem/Front Side HXs/Condenser ==
  Qcond : Inport
  AirMassFlow : Inport  Port=2
  AirTempRadOut : Inport  Port=3
  Add2 : Sum
  Add3 : Sum
  Gain4 : Gain  Gain=0.5
  LPF with IC2 : Subsystem  mask{wc=10, InitCond=EnvAirTemp, dataType=off}
      mask prompts: wc "Cutoff frequency, wc [rad/s]"; InitCond "Initial condition, InitCond [same as u]"; dataType "Enforce same input data type"
      mask TypeOptions wc: Cont LPF IC/wc
      mask TypeOptions InitCond: Initial Condition/Value
      mask TypeOptions dataType: Cont LPF IC/dataType
  Product4 : Product  Inputs=*/
  Product7 : Product
  Specific Heat Air 1 : Lookup_n-D  NumberOfTableDimensions=1  BreakpointsForDimension1=PlntThrAirCpBpt  Table=PlntThrAirCp  ExtrapMethod=Clip  UseLastTableValue=on  InternalRulePriority=Speed  RndMeth=Simplest
  div0protect - abs poly3 : autolibutils/div0protect - abs poly  thresh=.001  aMode=1
  AirTempOut : Outport
  wires:
  [AirTempRadOut] -> Add2/1
  Gain4/1 -> Specific Heat Air 1/1
  LPF with IC2/1(y) -> AirTempOut/1, [AirTempOut]
  Specific Heat Air 1/1 -> Product7/2
  Product4/1 -> Add2/2
  div0protect - abs poly3/1 -> Product4/2
  Add3/1 -> Gain4/1
  Add2/1 -> LPF with IC2/1(u)
  [AirTempOut] -> Add3/2
  Product7/1 -> div0protect - abs poly3/1
  AirTempRadOut/1 -> [AirTempRadOut], Add3/1
  Qcond/1 -> Product4/1
  AirMassFlow/1 -> Product7/1
